simulink model "bmgen_array_N3"  (R2014a)
settings: Solver=ode45  StartTime=0.0  StopTime=Tmax  RelTol=1e-3
PreLoadFcn:
  | N = 3;
  | addpath(['..', filesep, 'example', filesep, 'array']);
  | array_init;
values from neighbouring files (symbols this model uses):
  Tgrid = (1 / Fgrid)    (= 0.0166666666667)    [array_init.m]
  Ts = Tthd    (= 1.66666666667e-05)    [array_init.m]
  Tstartup = 3e-3    (= 0.003)    [array_init.m]
  Tswitch = [Tswitch; zeros(1,5)]    [array_init.m]
  Vgrid = (sqrt(2)*Vgridrms)    [array_init.m]
  Vref = 30    [array_init.m]
undefined symbols (not defined in the file or in its folder): Acarray, Aoarray, Bcarray, Boarray, Carray, Darray, Larray, Rarray
libraries: powerlib_meascontrol x3, module_switch x3
settings Model: Creator=Taylor  LastModifiedBy=tjohnson

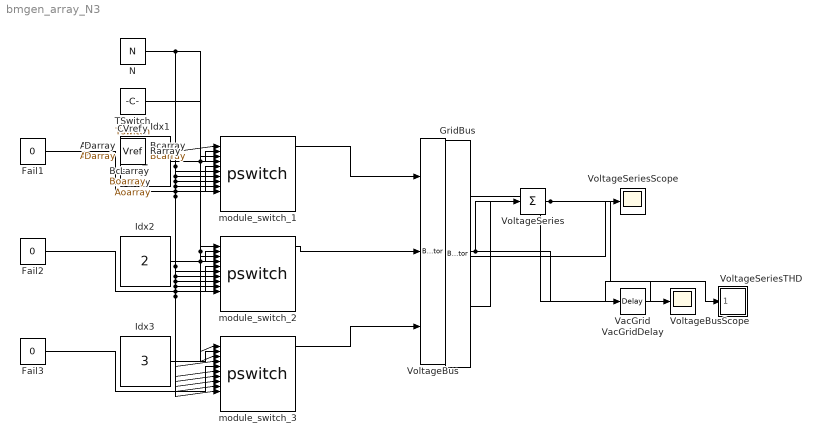
== system bmgen_array_N3 ==
  Acarray : Constant  Value=Acarray
  Aoarray : Constant  Value=Aoarray
  Bcarray : Constant  Value=Bcarray
  Boarray : Constant  Value=Boarray
  Carray : Constant  Value=Carray
  Darray : Constant  Value=Darray
  Fail1 : Constant  Value=0
  Fail2 : Constant  Value=0
  Fail3 : Constant  Value=0
  GridBus : BusCreator  Inputs=2
  Idx1 : Constant
  Idx2 : Constant  Value=2
  Idx3 : Constant  Value=3
  Larray : Constant  Value=Larray
  N : Constant  Value=N
  Rarray : Constant  Value=Rarray
  TSwitch : Constant  Value=Tswitch
  VacGrid : Sin  Amplitude=Vgrid  Frequency=2*pi/Tgrid
  VacGridDelay : TransportDelay  DelayTime=Tstartup
  VoltageBus : BusCreator  Inputs=N
  VoltageBusScope : Scope
  VoltageSeries : Sum  Inputs=+  SaturateOnIntegerOverflow=on  InputSameDT=on  OutDataTypeStr=Inherit: Same as first input
  VoltageSeriesScope : Scope
  VoltageSeriesTHD : Subsystem  VariantControl=Variant1
  Vref : Constant  Value=Vref
  module_switch_1 : module_switch/pswitch
  module_switch_2 : module_switch/pswitch
  module_switch_3 : module_switch/pswitch
  wires:
  VacGrid/1 -> VacGridDelay/1
  VacGridDelay/1 -> GridBus/1
  VoltageSeries/1 -> GridBus/2, VoltageSeriesTHD/1(In1)
  VoltageBus/1 -> VoltageSeries/1, VoltageBusScope/1
  GridBus/1 -> VoltageSeriesScope/1
  N/1 -> module_switch_2/1, module_switch_3/1, module_switch_1/1
  Idx1/1 -> module_switch_1/2
  Fail1/1 -> module_switch_1/5
  TSwitch/1 -> module_switch_2/3, module_switch_3/3, module_switch_1/3
  Darray/1 -> module_switch_2/4, module_switch_3/4, module_switch_1/4
  Acarray/1 -> module_switch_2/6, module_switch_3/6, module_switch_1/6
  Aoarray/1 -> module_switch_2/7, module_switch_3/7, module_switch_1/7
  Bcarray/1 -> module_switch_2/9, module_switch_3/9, module_switch_1/9
  Boarray/1 -> module_switch_2/8, module_switch_3/8, module_switch_1/8
  Vref/1 -> module_switch_2/10, module_switch_3/10, module_switch_1/10
  module_switch_1/1 -> VoltageBus/1
  Idx2/1 -> module_switch_2/2
  Fail2/1 -> module_switch_2/5
  module_switch_2/1 -> VoltageBus/2
  Idx3/1 -> module_switch_3/2
  Fail3/1 -> module_switch_3/5
  module_switch_3/1 -> VoltageBus/3

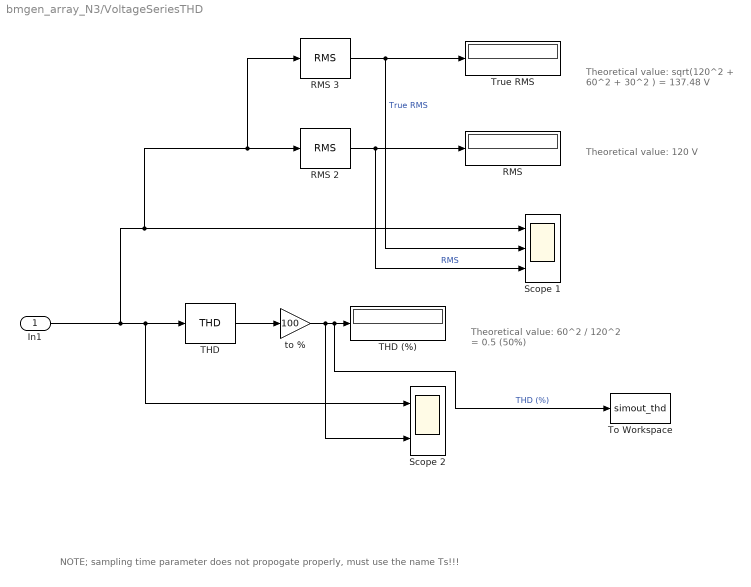
== system bmgen_array_N3/VoltageSeriesTHD ==
  note: NOTE; sampling time parameter does not propogate properly, must use the name Ts!!!
  note: Theoretical value:
      | 60^2 / 120^2 = 0.5  (50%)
  note: Theoretical value:
      | sqrt(120^2 + 60^2 + 30^2 )
      | = 137.48 V
  note: Theoretical value:
      | 120 V
  In1 : Inport
  RMS : Display
      settings: Format=bank
  RMS 2 : powerlib_meascontrol/Measurements/RMS  TrueRMS=off  Freq=Fgrid  RMSInit=Vgridrms  Ts=Ts
  RMS 3 : powerlib_meascontrol/Measurements/RMS  TrueRMS=on  Freq=Fgrid  RMSInit=Vgridrms  Ts=Ts
  Scope 1 : Scope  NumInputPorts=3
      settings: TimeRange=0.1  YMin=-250~50~50  YMax=250~150~150  SaveName=ScopeData2
  Scope 2 : Scope  NumInputPorts=2
      settings: TimeRange=0.0333333  YMin=-550~0  YMax=500~50
  THD : powerlib_meascontrol/Measurements/THD  Freq=Fgrid  Ts=Ts
  THD (%) : Display
      settings: Format=bank
  To Workspace : ToWorkspace  VariableName=simout_thd  SaveFormat=Timeseries  SampleTime=-1
  True RMS : Display
      settings: Format=bank
  to % : Gain  Gain=100  SampleTime=Ts
  wires:
  THD/1 -> to %/1
  to %/1 -> THD (%)/1, To Workspace/1, Scope 2/2  "THD (%)"
  In1/1 -> RMS 2/1, RMS 3/1, Scope 1/1, Scope 2/1, THD/1
  RMS 2/1 -> RMS/1, Scope 1/3  "RMS"
  RMS 3/1 -> True RMS/1, Scope 1/2  "True RMS"
